simulink model "VehiclePlantTestHarness"  (R2024a)
settings: configuration reference "standardSILConfiguraitonParams" (kept outside this file)
settings Model: Creator=jerem  LastModifiedBy=jerem
settings ConfigSetRef: SourceName=standardSILConfiguraitonParams  SourceLocation=Base Workspace

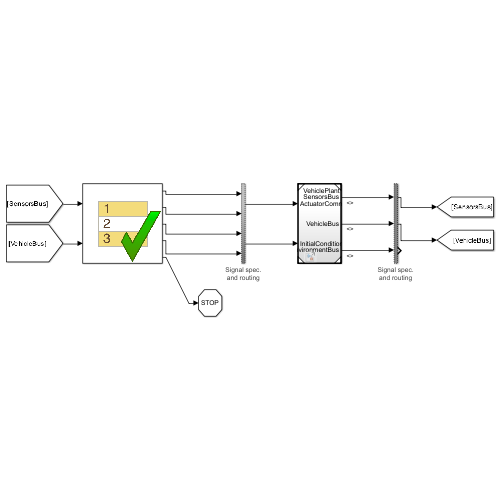
[thumbnail: Simulink's stored preview of the top-level diagram]
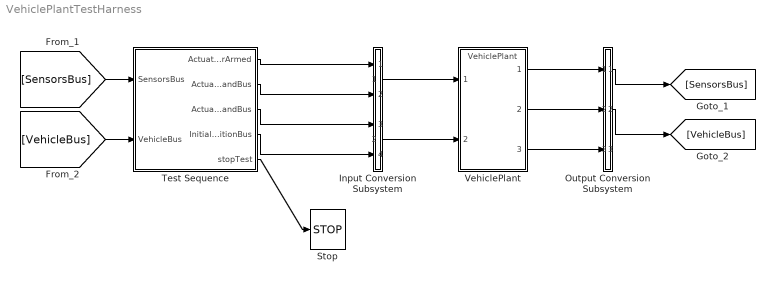
== system VehiclePlantTestHarness ==
  Input Conversion Subsystem : Subsystem  Tag=__SLT_ICS__  Description=|
      | Signal spec.
      | and routing
      settings: AttributesFormatString=%<Description>
  Output Conversion Subsystem : Subsystem  Tag=__SLT_OCS__  Description=|
      | Signal spec.
      | and routing
      mask init:
      | ICDictionary = get_param(bdroot, 'DataDictionary');
      | if isempty(ICDictionary)
      |    ICScope = Simulink.data.BaseWorkspace;
      | else
      |    ICScope = Simulink.data.DataDictionary(ICDictionary);
      | end
      | 
      | IC1 = Simulink.Bus.createMATLABStruct('SensorsBus', [], [1 1], ICScope);
      | IC2 = Simulink.Bus.createMATLABStruct('VehicleBus', [], [1 1], ICScope);
      | IC3 = Simulink.Bus.createMATLABStruct('EnvironmentBus', [], [1 1], ICScope);
      settings: AttributesFormatString=%<Description>
  Stop : Stop
  Test Sequence : Test Sequence  TreatAsAtomicUnit=on
  VehiclePlant : ModelReference  ModelNameDialog=VehiclePlant  SimulationMode=Normal  ModelReferenceVersion=1.27
  wires:
  Test Sequence/1(ActuatorCommandBus_controllerArmed) -> Input Conversion Subsystem/1(Inport_1)
  Test Sequence/2(ActuatorCommandBus_ServosCommandBus) -> Input Conversion Subsystem/2(Inport_2)
  Test Sequence/3(ActuatorCommandBus_EngineCommandBus) -> Input Conversion Subsystem/3(Inport_3)
  Test Sequence/4(InitialConditionBus) -> Input Conversion Subsystem/4(Inport_4)
  [SensorsBus] -> Test Sequence/1(SensorsBus)
  [VehicleBus] -> Test Sequence/2(VehicleBus)
  Output Conversion Subsystem/1(Outport_1) -> [SensorsBus]
  Output Conversion Subsystem/2(Outport_2) -> [VehicleBus]
  Test Sequence/5(stopTest) -> Stop/1
  VehiclePlant/1 -> Output Conversion Subsystem/1(Inport_1)
  VehiclePlant/2 -> Output Conversion Subsystem/2(Inport_2)
  VehiclePlant/3 -> Output Conversion Subsystem/3(Inport_3)
  Input Conversion Subsystem/1(Outport_1) -> VehiclePlant/1
  Input Conversion Subsystem/2(Outport_2) -> VehiclePlant/2

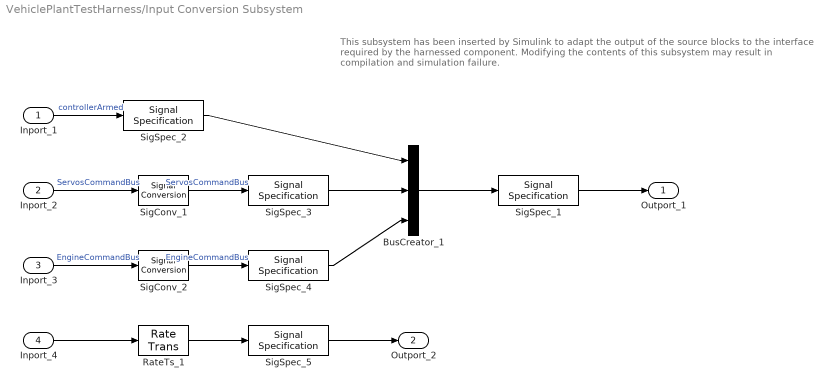
== system VehiclePlantTestHarness/Input Conversion Subsystem ==
  note: This subsystem has been inserted by Simulink to adapt the output of the source blocks to the interface required by the harnessed component.
      |  Modifying the contents of this subsystem may result in compilation and simulation failure.
  Inport_1 : Inport
  Inport_2 : Inport  Port=2
  Inport_3 : Inport  Port=3
  Inport_4 : Inport  Port=4
  BusCreator_1 : BusCreator  Inputs=3  OutDataTypeStr=Bus: ActuatorCommandBus
  RateTs_1 : RateTransition  OutPortSampleTime=0.004
  SigConv_1 : SignalConversion  ConversionOutput=Nonvirtual bus  OverrideOpt=off
  SigConv_2 : SignalConversion  ConversionOutput=Nonvirtual bus  OverrideOpt=off
  SigSpec_1 : SignalSpecification  OutDataTypeStr=Bus: ActuatorCommandBus  SampleTime=[-1, 0]
  SigSpec_2 : SignalSpecification  OutDataTypeStr=double  Dimensions=[1]  SampleTime=[-1, 0]
  SigSpec_3 : SignalSpecification  OutDataTypeStr=Bus: ServosCommandBus  Dimensions=[1]  SampleTime=[-1, 0]  BusOutputAsStruct=on
  SigSpec_4 : SignalSpecification  OutDataTypeStr=Bus: EngineCommandBus  Dimensions=[1]  SampleTime=[-1, 0]  BusOutputAsStruct=on
  SigSpec_5 : SignalSpecification  OutDataTypeStr=double  Dimensions=[1]  SampleTime=0.004
  Outport_1 : Outport
  Outport_2 : Outport  Port=2
  wires:
  SigSpec_1/1 -> Outport_1/1
  BusCreator_1/1 -> SigSpec_1/1
  SigSpec_2/1 -> BusCreator_1/1
  Inport_1/1 -> SigSpec_2/1  "controllerArmed"
  SigSpec_3/1 -> BusCreator_1/2
  SigConv_1/1 -> SigSpec_3/1  "ServosCommandBus"
  Inport_2/1 -> SigConv_1/1  "ServosCommandBus"
  SigSpec_4/1 -> BusCreator_1/3
  SigConv_2/1 -> SigSpec_4/1  "EngineCommandBus"
  Inport_3/1 -> SigConv_2/1  "EngineCommandBus"
  SigSpec_5/1 -> Outport_2/1
  RateTs_1/1 -> SigSpec_5/1
  Inport_4/1 -> RateTs_1/1

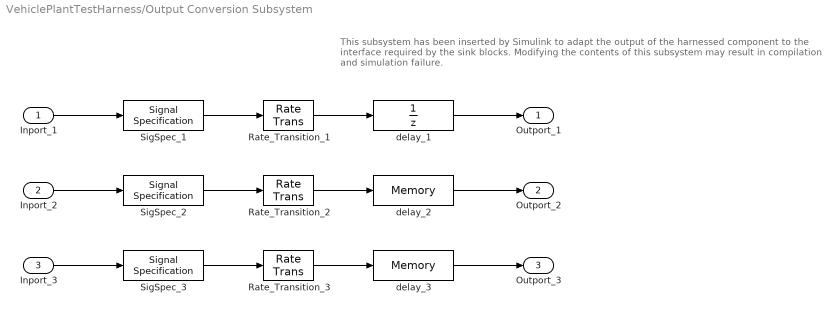
== system VehiclePlantTestHarness/Output Conversion Subsystem ==
  note: This subsystem has been inserted by Simulink to adapt the output of the harnessed component to the interface required by the sink blocks.
      |  Modifying the contents of this subsystem may result in compilation and simulation failure.
  Inport_1 : Inport
  Inport_2 : Inport  Port=2
  Inport_3 : Inport  Port=3
  Rate_Transition_1 : RateTransition  OutPortSampleTimeOpt=Inherit
  Rate_Transition_2 : RateTransition  OutPortSampleTimeOpt=Inherit
  Rate_Transition_3 : RateTransition  OutPortSampleTimeOpt=Inherit
  SigSpec_1 : SignalSpecification  OutDataTypeStr=Bus: SensorsBus  Dimensions=[1]  SampleTime=0.004
  SigSpec_2 : SignalSpecification  OutDataTypeStr=Bus: VehicleBus  Dimensions=[1]
  SigSpec_3 : SignalSpecification  OutDataTypeStr=Bus: EnvironmentBus  Dimensions=[1]
  delay_1 : UnitDelay  InitialCondition=IC1  SampleTime=-1
  delay_2 : Memory  InitialCondition=IC2
  delay_3 : Memory  InitialCondition=IC3
  Outport_1 : Outport
  Outport_2 : Outport  Port=2
  Outport_3 : Outport  Port=3
  wires:
  Inport_1/1 -> SigSpec_1/1
  SigSpec_1/1 -> Rate_Transition_1/1
  Rate_Transition_1/1 -> delay_1/1
  delay_1/1 -> Outport_1/1
  Inport_2/1 -> SigSpec_2/1
  SigSpec_2/1 -> Rate_Transition_2/1
  Rate_Transition_2/1 -> delay_2/1
  delay_2/1 -> Outport_2/1
  Inport_3/1 -> SigSpec_3/1
  SigSpec_3/1 -> Rate_Transition_3/1
  Rate_Transition_3/1 -> delay_3/1
  delay_3/1 -> Outport_3/1

== stateflow chart VehiclePlantTestHarness/Test Sequence ==
  state Error_Generator_1
    state Initialize
      %% Initialize data outputs.
      ActuatorCommandBus_controllerArmed = 0;
      ActuatorCommandBus_ServosCommandBus.ServosCommandF16Bus.cmdAileron_nd = 0;
      ActuatorCommandBus_ServosCommandBus.ServosCommandF16Bus.cmdElevator_nd = 0;
      ActuatorCommandBus_ServosCommandBus.ServosCommandF16Bus.cmdRudder_nd = 0;
      ActuatorCommandBus_ServosCommandBus.ServosCommandCustomAircraftBus.cmdControlSurfaceOne_nd = 0;
      ActuatorCommandBus_ServosCommandBus.ServosCommandCustomAircraftBus.cmdControlSurfaceTwo_nd = 0;
      ActuatorCommandBus_EngineCommandBus.cmdThrottle_unit = 0;
      InitialConditionBus = 0;
      stopTest = false;
    state step_1
      %% Initialize data outputs.
      ActuatorCommandBus_controllerArmed = 1;
      ActuatorCommandBus_EngineCommandBus.cmdThrottle_unit = 1;
      ActuatorCommandBus_ServosCommandBus.ServosCommandF16Bus.cmdElevator_nd = -0.15;
    state step_2
      %% Initialize data outputs.
      ActuatorCommandBus_ServosCommandBus.ServosCommandF16Bus.cmdElevator_nd = -0.03;
    state step_3
      ActuatorCommandBus_ServosCommandBus.ServosCommandF16Bus.cmdElevator_nd = -0.09;
    state EndTest
      stopTest = true;
    (default) -> Error_Generator_1.Initialize
    Error_Generator_1.Initialize -> Error_Generator_1.step_1 : [
        | true
        | ]
    Error_Generator_1.step_1 -> Error_Generator_1.step_2 : [
        | after(30,sec)
        | ]
    Error_Generator_1.step_2 -> Error_Generator_1.step_3 : [
        | after(100,sec)
        | ]
    Error_Generator_1.step_3 -> Error_Generator_1.EndTest : [
        | after(150,sec)
        | ]
  state Error_Generator_2
    state Initialize
      %% Initialize data outputs.
      ActuatorCommandBus_controllerArmed = 0;
      ActuatorCommandBus_ServosCommandBus.ServosCommandF16Bus.cmdAileron_nd = 0;
      ActuatorCommandBus_ServosCommandBus.ServosCommandF16Bus.cmdElevator_nd = 0;
      ActuatorCommandBus_ServosCommandBus.ServosCommandF16Bus.cmdRudder_nd = 0;
      ActuatorCommandBus_ServosCommandBus.ServosCommandCustomAircraftBus.cmdControlSurfaceOne_nd = 0;
      ActuatorCommandBus_ServosCommandBus.ServosCommandCustomAircraftBus.cmdControlSurfaceTwo_nd = 0;
      ActuatorCommandBus_EngineCommandBus.cmdThrottle_unit = 0;
      InitialConditionBus = 0;
      stopTest = false;
    state step_1
      %% Initialize data outputs.
      ActuatorCommandBus_controllerArmed = 1;
      ActuatorCommandBus_EngineCommandBus.cmdThrottle_unit = 1;
      ActuatorCommandBus_ServosCommandBus.ServosCommandF16Bus.cmdElevator_nd = -0.15;
    state step_2
      %% Initialize data outputs.
      ActuatorCommandBus_ServosCommandBus.ServosCommandF16Bus.cmdElevator_nd = -0.03;
    state step_3
      ActuatorCommandBus_ServosCommandBus.ServosCommandF16Bus.cmdElevator_nd = -0.05;
    state EndTest
      stopTest = true;
    (default) -> Error_Generator_2.Initialize
    Error_Generator_2.Initialize -> Error_Generator_2.step_1 : [
        | true
        | ]
    Error_Generator_2.step_1 -> Error_Generator_2.step_2 : [
        | after(30,sec)
        | ]
    Error_Generator_2.step_2 -> Error_Generator_2.step_3 : [
        | after(100,sec)
        | ]
    Error_Generator_2.step_3 -> Error_Generator_2.EndTest : [
        | after(150,sec)
        | ]
  state Error_Generator_3
    state Initialize
      %% Initialize data outputs.
      ActuatorCommandBus_controllerArmed = 0;
      ActuatorCommandBus_ServosCommandBus.ServosCommandF16Bus.cmdAileron_nd = 0;
      ActuatorCommandBus_ServosCommandBus.ServosCommandF16Bus.cmdElevator_nd = 0;
      ActuatorCommandBus_ServosCommandBus.ServosCommandF16Bus.cmdRudder_nd = 0;
      ActuatorCommandBus_ServosCommandBus.ServosCommandCustomAircraftBus.cmdControlSurfaceOne_nd = 0;
      ActuatorCommandBus_ServosCommandBus.ServosCommandCustomAircraftBus.cmdControlSurfaceTwo_nd = 0;
      ActuatorCommandBus_EngineCommandBus.cmdThrottle_unit = 0;
      InitialConditionBus = 0;
      stopTest = false;
    state step_1
      %% Initialize data outputs.
      ActuatorCommandBus_controllerArmed = 1;
      ActuatorCommandBus_EngineCommandBus.cmdThrottle_unit = 1;
      ActuatorCommandBus_ServosCommandBus.ServosCommandF16Bus.cmdElevator_nd = -0.15;
    state step_2
      %% Initialize data outputs.
      ActuatorCommandBus_ServosCommandBus.ServosCommandF16Bus.cmdElevator_nd = -0.03;
    state step_3
      ActuatorCommandBus_ServosCommandBus.ServosCommandF16Bus.cmdElevator_nd = -0.03;
    state EndTest
      stopTest = true;
    (default) -> Error_Generator_3.Initialize
    Error_Generator_3.Initialize -> Error_Generator_3.step_1 : [
        | true
        | ]
    Error_Generator_3.step_1 -> Error_Generator_3.step_2 : [
        | after(30,sec)
        | ]
    Error_Generator_3.step_2 -> Error_Generator_3.step_3 : [
        | after(100,sec)
        | ]
    Error_Generator_3.step_3 -> Error_Generator_3.EndTest : [
        | after(150,sec)
        | ]
  (default) -> Error_Generator_1 [order 1] : [Active_Scenario_Index == 1]
  (default) -> Error_Generator_2 [order 2] : [Active_Scenario_Index == 2]
  (default) -> Error_Generator_3 [order 3] : {assert(Active_Scenario_Index == 3,'The value of Scenario Parameter ''Active_Scenario_Index'' is not valid. Use the index of the scenario to specify it.')}
  data: SensorsBus input Bus: SensorsBus size=[1]; VehicleBus input Bus: VehicleBus size=[1]; ActuatorCommandBus_controllerArmed output double size=[1]; ActuatorCommandBus_ServosCommandBus output Bus: ServosCommandBus size=[1]; ActuatorCommandBus_EngineCommandBus output Bus: EngineCommandBus size=[1]; InitialConditionBus output double size=[1]; stopTest output; Active_Scenario_Index parameter =3
